simulink subsystem "MIMO_attitude_adaptive_smc"  (R2023b)
settings: Solver=VariableStepAuto  StartTime=0.0  StopTime=10.0  RelTol=1e-3
undefined symbols (not defined in the file or in its folder): GHV_cfg
libraries: aerolibadyn x1
settings Model: Creator=Admin  LastModifiedBy=Admin

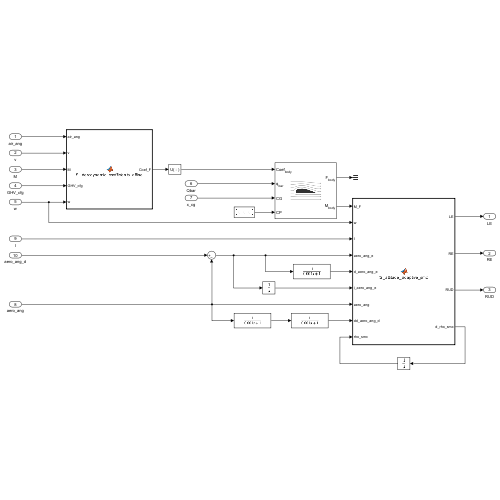
[thumbnail: Simulink's stored preview of the top-level diagram]
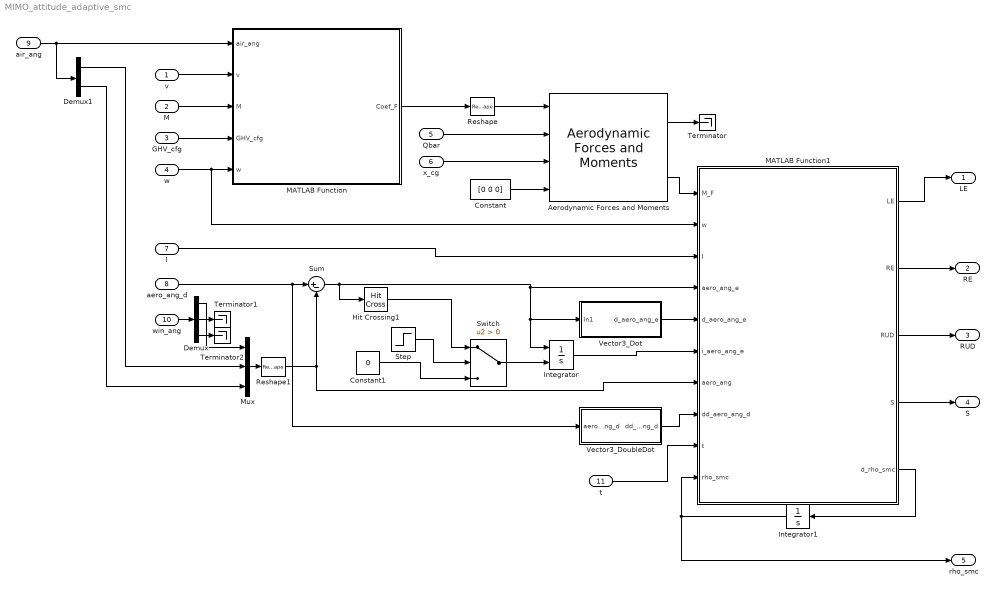
== system MIMO_attitude_adaptive_smc ==
  v : Inport
  M : Inport  Port=2
  GHV_cfg : Inport  Port=3
  w : Inport  Port=4
  Qbar : Inport  Port=5
  x_cg : Inport  Port=6
  I : Inport  Port=7
  aero_ang_d : Inport  Port=8
  air_ang : Inport  Port=9
  win_ang : Inport  Port=10
  t : Inport  Port=11
  "Aerodynamic Forces and Moments " : aerolibadyn/Aerodynamic Forces and Moments   inputAxes=Body  outputForceAxes=Body  outputMomentAxes=Body  S=GHV_cfg.s_ref  b=GHV_cfg.b_ref  cbar=GHV_cfg.c_ref
  Constant : Constant  Value=[0 0 0]
  Constant1 : Constant  Value=0
  Demux : Demux  Outputs=3
  Demux1 : Demux  Outputs=2
  Hit Crossing1 : HitCross  HitCrossingDirection=falling
  Integrator : Integrator  ExternalReset=either
  Integrator1 : Integrator  InitialCondition=[0;0;0]
  MATLAB Function : MATLAB Function  TreatAsAtomicUnit=on
  MATLAB Function1 : MATLAB Function  TreatAsAtomicUnit=on
  Mux : Mux  Inputs=3
  Reshape : Reshape
  Reshape1 : Reshape  OutputDimensionality=Column vector (2-D)
  Step : Step  Time=15  Before=1  After=0  SampleTime=0
  Sum : Sum  Inputs=|+-
  Switch : Switch  Criteria=u2 > Threshold  SaturateOnIntegerOverflow=off  InputSameDT=off
  Terminator : Terminator
  Terminator1 : Terminator
  Terminator2 : Terminator
  Vector3_Dot : Subsystem
  Vector3_DoubleDot : Subsystem
  LE : Outport
  RE : Outport  Port=2
  RUD : Outport  Port=3
  S : Outport  Port=4
  rho_smc : Outport  Port=5
  wires:
  v/1 -> MATLAB Function/2(v)
  w/1 -> MATLAB Function1/2(w), MATLAB Function/5(w)
  M/1 -> MATLAB Function/3(M)
  GHV_cfg/1 -> MATLAB Function/4(GHV_cfg)
  MATLAB Function/1(Coef_F) -> Reshape/1
  Reshape/1 -> "Aerodynamic Forces and Moments "/1
  Qbar/1 -> "Aerodynamic Forces and Moments "/2
  x_cg/1 -> "Aerodynamic Forces and Moments "/3
  Constant/1 -> "Aerodynamic Forces and Moments "/4
  "Aerodynamic Forces and Moments "/1 -> Terminator/1
  "Aerodynamic Forces and Moments "/2 -> MATLAB Function1/1(M_F)
  I/1 -> MATLAB Function1/3(I)
  Mux/1 -> Reshape1/1
  aero_ang_d/1 -> Sum/1, Vector3_DoubleDot/1(aero_ang_d)
  Sum/1 -> Hit Crossing1/1, MATLAB Function1/4(aero_ang_e), Vector3_Dot/1(In1), Integrator/1
  Integrator/1 -> MATLAB Function1/6(i_aero_ang_e)
  MATLAB Function1/5(d_rho_smc) -> Integrator1/1
  Integrator1/1 -> rho_smc/1, MATLAB Function1/10(rho_smc)
  Vector3_DoubleDot/1(dd_aero_ang_d) -> MATLAB Function1/8(dd_aero_ang_d)
  MATLAB Function1/1(LE) -> LE/1
  MATLAB Function1/2(RE) -> RE/1
  MATLAB Function1/3(RUD) -> RUD/1
  air_ang/1 -> MATLAB Function/1(air_ang), Demux1/1
  win_ang/1 -> Demux/1
  Demux/3 -> Terminator2/1
  Demux/2 -> Terminator1/1
  Demux/1 -> Mux/1
  Demux1/2 -> Mux/3
  Demux1/1 -> Mux/2
  Reshape1/1 -> Sum/2, MATLAB Function1/7(aero_ang)
  Vector3_Dot/1(d_aero_ang_e) -> MATLAB Function1/5(d_aero_ang_e)
  MATLAB Function1/4(S) -> S/1
  Hit Crossing1/1 -> Switch/1
  Step/1 -> Switch/2
  Constant1/1 -> Switch/3
  Switch/1 -> Integrator/2
  t/1 -> MATLAB Function1/9(t)

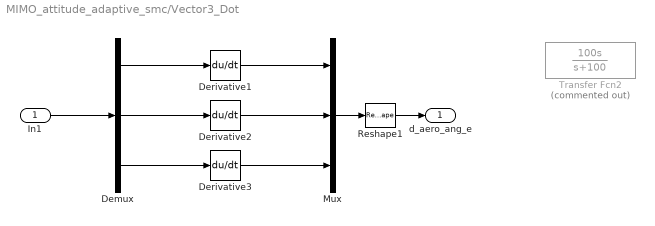
== system MIMO_attitude_adaptive_smc/Vector3_Dot ==
  In1 : Inport
  Demux : Demux  Outputs=3
  Derivative1 : Derivative
  Derivative2 : Derivative
  Derivative3 : Derivative
  Mux : Mux  Inputs=3
  Reshape1 : Reshape  OutputDimensionality=Column vector (2-D)
  Transfer Fcn2 : TransferFcn  Commented=on  Numerator=[100 0]  Denominator=[1 100]
  d_aero_ang_e : Outport
  wires:
  Derivative3/1 -> Mux/3
  Derivative2/1 -> Mux/2
  Derivative1/1 -> Mux/1
  Reshape1/1 -> d_aero_ang_e/1
  Mux/1 -> Reshape1/1
  Demux/3 -> Derivative3/1
  Demux/1 -> Derivative1/1
  Demux/2 -> Derivative2/1
  In1/1 -> Demux/1

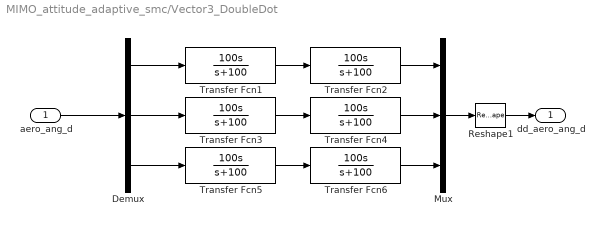
== system MIMO_attitude_adaptive_smc/Vector3_DoubleDot ==
  aero_ang_d : Inport
  Demux : Demux  Outputs=3
  Mux : Mux  Inputs=3
  Reshape1 : Reshape  OutputDimensionality=Column vector (2-D)
  Transfer Fcn{1..6} (6 alike) : TransferFcn  Numerator=[100 0]  Denominator=[1 100]
  dd_aero_ang_d : Outport
  wires:
  Reshape1/1 -> dd_aero_ang_d/1
  Mux/1 -> Reshape1/1
  Transfer Fcn2/1 -> Mux/1
  Transfer Fcn6/1 -> Mux/3
  Transfer Fcn4/1 -> Mux/2
  Demux/3 -> Transfer Fcn5/1
  Demux/1 -> Transfer Fcn1/1
  Demux/2 -> Transfer Fcn3/1
  Transfer Fcn5/1 -> Transfer Fcn6/1
  Transfer Fcn3/1 -> Transfer Fcn4/1
  aero_ang_d/1 -> Demux/1
  Transfer Fcn1/1 -> Transfer Fcn2/1

== matlab function MIMO_attitude_adaptive_smc/MATLAB Function ==
  data: air_ang input; Coef_F output; v input; M input; GHV_cfg input; w input
function Coef_F = S_Aerodynamic_coefficients_affine(air_ang, v, M, GHV_cfg, w)

    Coef_F = Aerodynamic_coefficients_affine(air_ang, v, w, M, GHV_cfg);

end

== matlab function MIMO_attitude_adaptive_smc/MATLAB Function1 ==
  data: M_F input; w input; I input; LE output; aero_ang_e input; d_aero_ang_e input; i_aero_ang_e input; aero_ang input; dd_aero_ang_d input; t input; rho_smc input; RE output; RUD output; S output; d_rho_smc output
function  [LE, RE, RUD, S, d_rho_smc] = S_attitude_adaptive_smc(M_F, w, I, aero_ang_e, d_aero_ang_e, i_aero_ang_e, aero_ang, dd_aero_ang_d, t, rho_smc)
    
        d_rho_smc = zeros(3, 1); %#ok<PREALL>
     [LE, RE, RUD, d_rho_smc, S] = attitude_adaptive_smc(I, w, aero_ang, dd_aero_ang_d, aero_ang_e, d_aero_ang_e, i_aero_ang_e, rho_smc, M_F,t);

end
